simulink model "Fautlframework"  (R2014a)
settings: Solver=FixedStepDiscrete  StartTime=0.0  StopTime=SimLength  FixedStep=sample_time  RelTol=1e-3
InitFcn:
  | sample_time = 0.05
settings Model: Creator=georg  LastModifiedBy=root

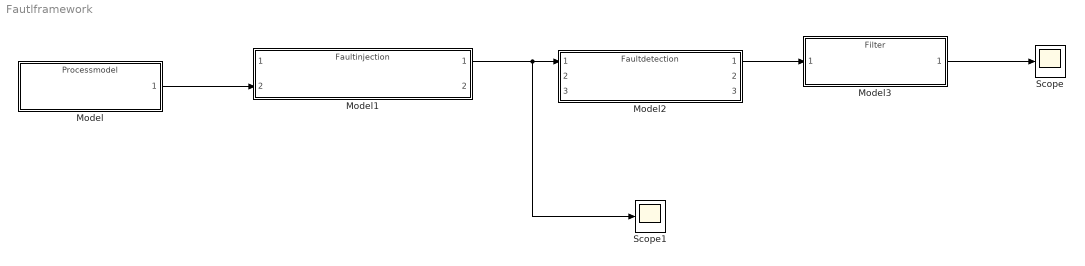
== system Fautlframework ==
  Model : ModelReference  ModelNameDialog=Processmodel  SimulationMode=Normal  ModelReferenceVersion=1.8  CopyOfModelName=Processmodel  DefaultDataLogging=on
  Model1 : ModelReference  ModelNameDialog=Faultinjection  SimulationMode=Normal  ModelReferenceVersion=1.6  CopyOfModelName=Faultinjection  DefaultDataLogging=on
  Model2 : ModelReference  ModelNameDialog=Faultdetection  SimulationMode=Normal  ModelReferenceVersion=1.35  CopyOfModelName=Faultdetection  DefaultDataLogging=on
  Model3 : ModelReference  ModelNameDialog=Filter  SimulationMode=Normal  ModelReferenceVersion=1.3  CopyOfModelName=Filter  DefaultDataLogging=on
  Scope : Scope
  Scope1 : Scope
  wires:
  Model/1 -> Model1/2
  Model1/1 -> Scope1/1, Model2/1
  Model2/1 -> Model3/1
  Model3/1 -> Scope/1
